simulink model "second_24_02_25_FRANCO"  (R2024a)
settings: Solver=VariableStepAuto  StartTime=0.0  StopTime=inf  FixedStep=1e-3  MaxStep=100e-6  RelTol=0.1e-3
values from neighbouring files (symbols this model uses):
  f = 5000    [second_parameters.m]
  l = 10e-3    (= 0.01)    [second_parameters.m]
  phi = atan(f*2*pi*l/r)    [second_parameters.m]
  r = 10    [second_parameters.m]
  z = sqrt(r^2+(2*pi*f*l)^2)    [second_parameters.m]
libraries: simulink x4, simulink_extras x1
settings Model: Creator=claudio.rossi  LastModifiedBy=s0001205361
settings OptimizationCC: ReuseModelBlockBuffer=off
settings RTWCC: GPUComputeCapability=3.5

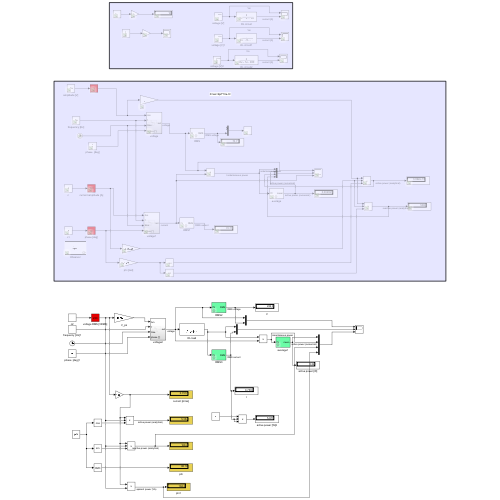
[thumbnail: Simulink's stored preview of the top-level diagram]
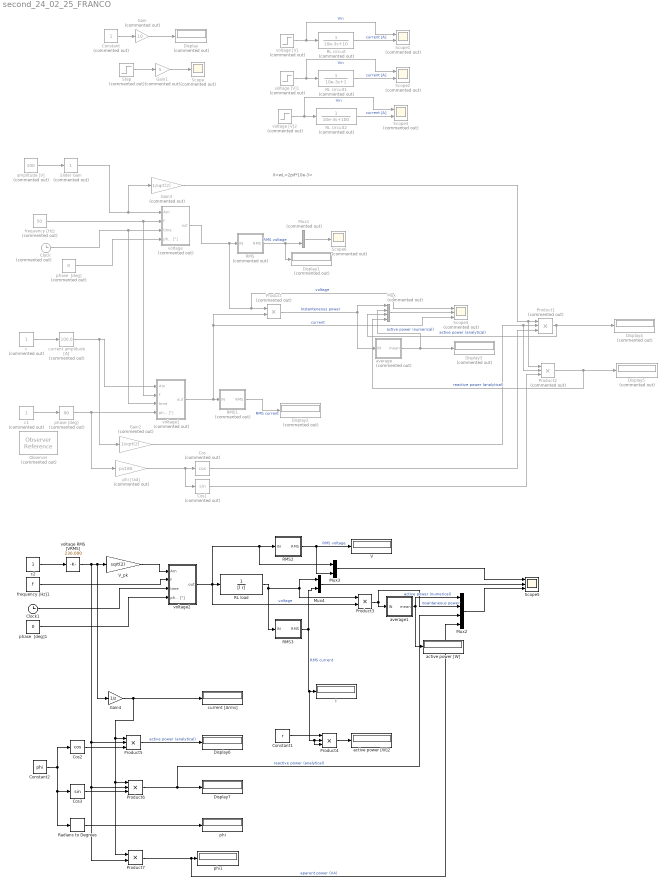
== system second_24_02_25_FRANCO ==
  note: X=wL=2pif*10e-3=
  Clock : Clock  Commented=on
  Clock1 : Clock
  Constant : Constant  Commented=on
  Constant1 : Constant  Value=r
  Constant2 : Constant  Value=phi
  Cos : Trigonometry  Commented=on  Operator=cos
  Cos1 : Trigonometry  Commented=on
  Cos2 : Trigonometry  Operator=cos
  Cos3 : Trigonometry
  Display{,1..5} (6 alike) : Display  Commented=on
  Display6 : Display
  Display7 : Display
  Gain : Gain  Commented=on  Gain=10
  Gain1 : Gain  Commented=on  Gain=5
  Gain2 : Gain  Commented=on  Gain=1/sqrt(2)
  Gain3 : Gain  Commented=on  Gain=1/sqrt(2)
  Gain4 : Gain  Gain=1/z
  I : Display
  Mux : Mux  Commented=on
  Mux1 : Mux  Commented=on  Inputs=2
  Mux2 : Mux
  Mux3 : Mux  Inputs=2
  Mux4 : Mux  Inputs=2
  Observer : ObserverReference  Commented=on  ObserverModelName=second_24_02_25_FRANCO_Observer1
  Product : Product  Commented=on
  Product1 : Product  Commented=on  Inputs=3
  Product2 : Product  Commented=on  Inputs=3
  Product3 : Product
  Product4 : Product  Inputs=3
  Product5 : Product  Inputs=3
  Product6 : Product  Inputs=3
  Product7 : Product
  RL circuit : TransferFcn  Commented=on  Denominator=[10e-3 10]
  RL circuit1 : TransferFcn  Commented=on  Denominator=[10e-3 1]
  RL circuit2 : TransferFcn  Commented=on  Denominator=[10e-3 100]
  RL load : TransferFcn  Denominator=[l r]
  RMS : Subsystem  Commented=on  mask{period=20e-3}
      mask prompts: period "period [s]"
      mask DialogControl DescTextVar Prompt: calculates the RMS of a periodic function with period specified here
  RMS1 : Subsystem  Commented=on  mask{period=20e-3}
      mask prompts: period "period [s]"
      mask DialogControl DescTextVar Prompt: calculates the RMS of a periodic function with period specified here
  RMS2 : Subsystem  mask{period=1/f}
      mask prompts: period "period [s]"
      mask DialogControl DescTextVar Prompt: calculates the RMS of a periodic function with period specified here
  RMS3 : Subsystem  mask{period=1/f}
      mask prompts: period "period [s]"
      mask DialogControl DescTextVar Prompt: calculates the RMS of a periodic function with period specified here
  Radians to Degrees : simulink_extras/Transformations/Radians to Degrees
  Scope : Scope  Commented=on
  Scope1 : Scope  Commented=on  NumInputPorts=2
  Scope2 : Scope  Commented=on  NumInputPorts=2
  Scope3 : Scope  Commented=on  NumInputPorts=2
  Scope4 : Scope  Commented=on  NumInputPorts=3
  Scope5 : Scope  NumInputPorts=3
  Scope6 : Scope  Commented=on
  Slider Gain : simulink/Math Operations/Slider Gain  Commented=on  gain=1  low=0  high=2
  Step : Step  Commented=on  SampleTime=0
  V : Display
  V_pk : Gain  Gain=sqrt(2)
  active power [W] : Display
  active power [W]2 : Display
  amplitude [V] : Constant  Commented=on  Value=100
  average : Subsystem  Commented=on  mask{period=20}
      mask prompts: period "period [s]"
  average1 : Subsystem  mask{period=20}
      mask prompts: period "period [s]"
  c : Constant  Commented=on
  c1 : Constant  Commented=on
  c2 : Constant
  current [Arms] : Display
  current amplitude [A] : simulink/Math Operations/Slider Gain  Commented=on  gain=100.0  low=0  high=100
  frequency [Hz] : Constant  Commented=on  Value=50
  frequency [Hz]1 : Constant  Value=f
  phase  [deg] : Constant  Commented=on  Value=0
  phase  [deg]1 : Constant  Value=0
  phase [deg] : simulink/Math Operations/Slider Gain  Commented=on  gain=90  low=-180  high=180
  phi : Display
  phi [rad] : Gain  Commented=on  Gain=pi/180
  phi1 : Display
  voltage : Subsystem  Commented=on
  voltage RMS [VRMS] : simulink/Math Operations/Slider Gain  gain=230.000  low=0  high=230
  voltage [V] : Step  Commented=on  After=100  SampleTime=0
  voltage [V]1 : Step  Commented=on  After=100  SampleTime=0
  voltage [V]2 : Step  Commented=on  After=100  SampleTime=0
  voltage1 : Subsystem  Commented=on
  voltage2 : Subsystem
  wires:
  Constant/1 -> Gain/1
  Step/1 -> Gain1/1
  Gain/1 -> Display/1
  Gain1/1 -> Scope/1
  voltage [V]/1 -> Scope1/1, RL circuit/1  "Vin"
  RL circuit/1 -> Scope1/2  "current [A]"
  RL circuit1/1 -> Scope2/2  "current [A]"
  voltage [V]1/1 -> RL circuit1/1, Scope2/1  "Vin"
  voltage [V]2/1 -> Scope3/1, RL circuit2/1  "Vin"
  RL circuit2/1 -> Scope3/2  "current [A]"
  amplitude [V]/1 -> Slider Gain/1
  frequency [Hz]/1 -> voltage1/2(f), voltage/2(f)
  Clock/1 -> voltage1/3(time), voltage/3(time)
  phase  [deg]/1 -> voltage/4(phase [°])
  voltage/1(out) -> Scope4/1, Product/1, RMS/1(IN)  "voltage"
  Slider Gain/1 -> Gain3/1, voltage/1(Am)
  Mux1/1 -> Scope6/1
  RMS/1(RMS) -> Display1/1, Mux1/2  "RMS voltage"
  current amplitude [A]/1 -> Gain2/1, voltage1/1(Am)
  c1/1 -> phase [deg]/1
  c/1 -> current amplitude [A]/1
  phase [deg]/1 -> phi [rad]/1, voltage1/4(phase [°])
  voltage1/1(out) -> Scope4/3, Product/2, RMS1/1(IN)  "current"
  RMS1/1(RMS) -> Display2/1  "RMS current"
  Product/1 -> average/1(IN), Mux/1  "Instanteneous power"
  average/1(mean) -> Mux/2, Display3/1  "active power (numerical)"
  Mux/1 -> Scope4/2
  Gain3/1 -> Product2/1, Product1/1
  Gain2/1 -> Product2/2, Product1/2
  phi [rad]/1 -> Cos1/1, Cos/1
  Cos/1 -> Product1/3
  Product1/1 -> Mux/3, Display4/1  "active power (analytical)"
  Product2/1 -> Mux/4, Display5/1  "reactive power (analytical)"
  Cos1/1 -> Product2/3
  voltage RMS [VRMS]/1 -> V_pk/1, Gain4/1, Product7/2, Product6/2, Product5/2
  phase  [deg]1/1 -> voltage2/4(phase [°])
  Clock1/1 -> voltage2/3(time)
  frequency [Hz]1/1 -> voltage2/2(f)
  c2/1 -> voltage RMS [VRMS]/1
  V_pk/1 -> voltage2/1(Am)
  voltage2/1(out) -> Product3/2, Mux3/1, RMS2/1(IN), RL load/1  "voltage"
  RL load/1 -> RMS3/1(IN), Product3/1, Mux4/1
  Mux2/1 -> Scope5/3
  RMS2/1(RMS) -> Mux3/2, V/1  "RMS voltage"
  RMS3/1(RMS) -> Mux4/2, Product4/3, Product4/2, I/1  "RMS current"
  Mux3/1 -> Scope5/1
  Mux4/1 -> Scope5/2
  Product3/1 -> Mux2/2, average1/1(IN)  "insantaneous power"
  average1/1(mean) -> Mux2/1, active power [W]/1  "active power (numerical)"
  Constant1/1 -> Product4/1
  Product4/1 -> active power [W]2/1
  Product6/1 -> Mux2/3, Display7/1  "reactive power (analytical)"
  Product5/1 -> Display6/1  "active power (analytical)"
  Gain4/1 -> Product5/1, Product7/1, Product6/1, current [Arms]/1
  Cos2/1 -> Product5/3
  Cos3/1 -> Product6/3
  Constant2/1 -> Radians to Degrees/1, Cos3/1, Cos2/1
  Radians to Degrees/1 -> phi/1
  Product7/1 -> Mux2/4, phi1/1  "aparent power (VA)"

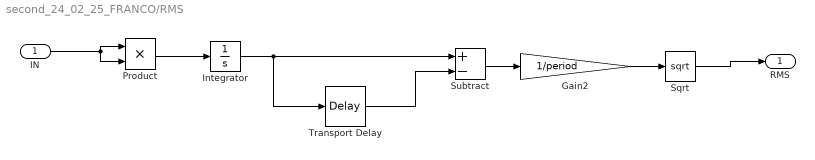
== system second_24_02_25_FRANCO/RMS ==
  IN : Inport
  Gain2 : Gain  Gain=1/period
  Integrator : Integrator
  Product : Product
  Sqrt : Sqrt
  Subtract : Sum  Inputs=+-
  Transport Delay : TransportDelay  DelayTime=period
  RMS : Outport
  wires:
  Transport Delay/1 -> Subtract/2
  Subtract/1 -> Gain2/1
  Integrator/1 -> Subtract/1, Transport Delay/1
  IN/1 -> Product/1, Product/2
  Product/1 -> Integrator/1
  Gain2/1 -> Sqrt/1
  Sqrt/1 -> RMS/1

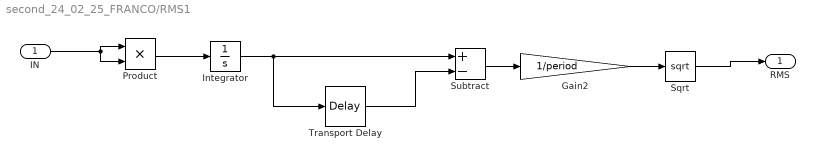
== system second_24_02_25_FRANCO/RMS1 ==
  IN : Inport
  Gain2 : Gain  Gain=1/period
  Integrator : Integrator
  Product : Product
  Sqrt : Sqrt
  Subtract : Sum  Inputs=+-
  Transport Delay : TransportDelay  DelayTime=period
  RMS : Outport
  wires:
  Sqrt/1 -> RMS/1
  Gain2/1 -> Sqrt/1
  Product/1 -> Integrator/1
  IN/1 -> Product/2, Product/1
  Integrator/1 -> Transport Delay/1, Subtract/1
  Subtract/1 -> Gain2/1
  Transport Delay/1 -> Subtract/2

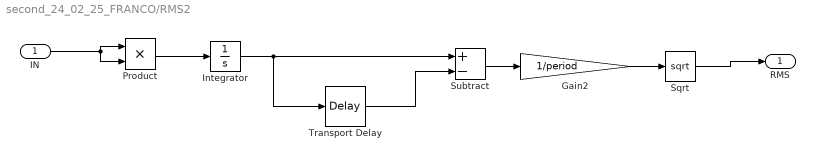
== system second_24_02_25_FRANCO/RMS2 ==
  IN : Inport
  Gain2 : Gain  Gain=1/period
  Integrator : Integrator
  Product : Product
  Sqrt : Sqrt
  Subtract : Sum  Inputs=+-
  Transport Delay : TransportDelay  DelayTime=period
  RMS : Outport
  wires:
  Sqrt/1 -> RMS/1
  Gain2/1 -> Sqrt/1
  Product/1 -> Integrator/1
  IN/1 -> Product/2, Product/1
  Integrator/1 -> Transport Delay/1, Subtract/1
  Subtract/1 -> Gain2/1
  Transport Delay/1 -> Subtract/2

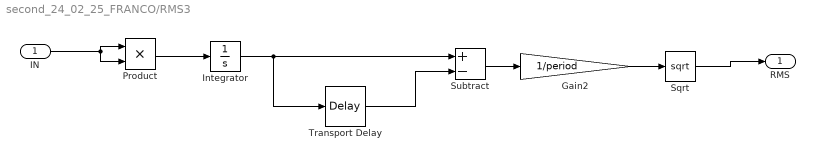
== system second_24_02_25_FRANCO/RMS3 ==
  IN : Inport
  Gain2 : Gain  Gain=1/period
  Integrator : Integrator
  Product : Product
  Sqrt : Sqrt
  Subtract : Sum  Inputs=+-
  Transport Delay : TransportDelay  DelayTime=period
  RMS : Outport
  wires:
  Transport Delay/1 -> Subtract/2
  Subtract/1 -> Gain2/1
  Integrator/1 -> Subtract/1, Transport Delay/1
  IN/1 -> Product/1, Product/2
  Product/1 -> Integrator/1
  Gain2/1 -> Sqrt/1
  Sqrt/1 -> RMS/1

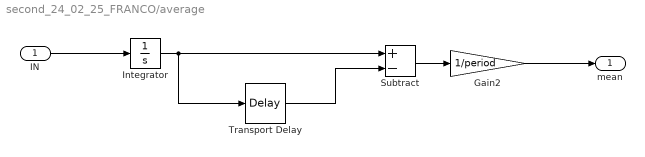
== system second_24_02_25_FRANCO/average ==
  IN : Inport
  Gain2 : Gain  Gain=1/period
  Integrator : Integrator
  Subtract : Sum  Inputs=+-
  Transport Delay : TransportDelay  DelayTime=period
  mean : Outport
  wires:
  IN/1 -> Integrator/1
  Transport Delay/1 -> Subtract/2
  Subtract/1 -> Gain2/1
  Gain2/1 -> mean/1
  Integrator/1 -> Subtract/1, Transport Delay/1

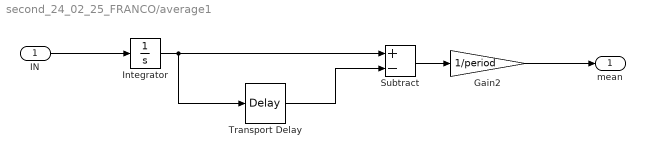
== system second_24_02_25_FRANCO/average1 ==
  IN : Inport
  Gain2 : Gain  Gain=1/period
  Integrator : Integrator
  Subtract : Sum  Inputs=+-
  Transport Delay : TransportDelay  DelayTime=period
  mean : Outport
  wires:
  Integrator/1 -> Transport Delay/1, Subtract/1
  Gain2/1 -> mean/1
  Subtract/1 -> Gain2/1
  Transport Delay/1 -> Subtract/2
  IN/1 -> Integrator/1

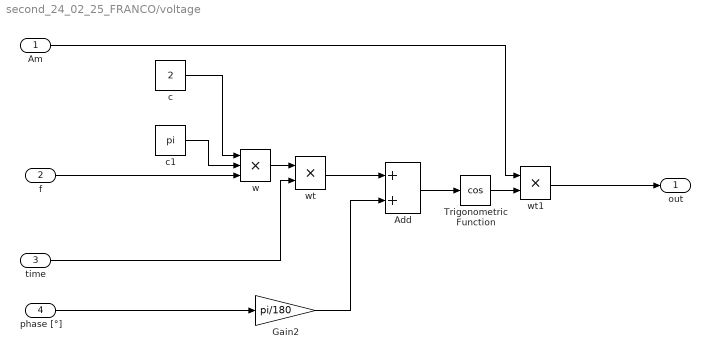
== system second_24_02_25_FRANCO/voltage ==
  Am : Inport
  f : Inport  Port=2
  time : Inport  Port=3
  phase [°] : Inport  Port=4
  Add : Sum
  Gain2 : Gain  Gain=pi/180
  Trigonometric Function : Trigonometry  Operator=cos
  c : Constant  Value=2
  c1 : Constant  Value=pi
  w : Product  Inputs=3
  wt : Product
  wt1 : Product
  out : Outport
  wires:
  wt/1 -> Add/1
  Add/1 -> Trigonometric Function/1
  phase [°]/1 -> Gain2/1
  c/1 -> w/1
  w/1 -> wt/1
  Trigonometric Function/1 -> wt1/2
  c1/1 -> w/2
  Gain2/1 -> Add/2
  wt1/1 -> out/1
  f/1 -> w/3
  time/1 -> wt/2
  Am/1 -> wt1/1

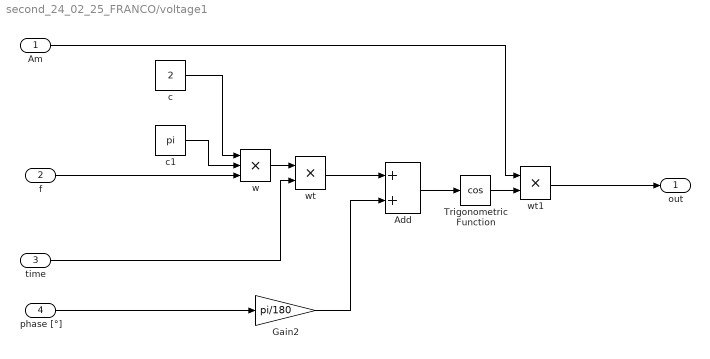
== system second_24_02_25_FRANCO/voltage1 ==
  Am : Inport
  f : Inport  Port=2
  time : Inport  Port=3
  phase [°] : Inport  Port=4
  Add : Sum
  Gain2 : Gain  Gain=pi/180
  Trigonometric Function : Trigonometry  Operator=cos
  c : Constant  Value=2
  c1 : Constant  Value=pi
  w : Product  Inputs=3
  wt : Product
  wt1 : Product
  out : Outport
  wires:
  Am/1 -> wt1/1
  time/1 -> wt/2
  f/1 -> w/3
  wt1/1 -> out/1
  Gain2/1 -> Add/2
  c1/1 -> w/2
  Trigonometric Function/1 -> wt1/2
  w/1 -> wt/1
  c/1 -> w/1
  phase [°]/1 -> Gain2/1
  Add/1 -> Trigonometric Function/1
  wt/1 -> Add/1

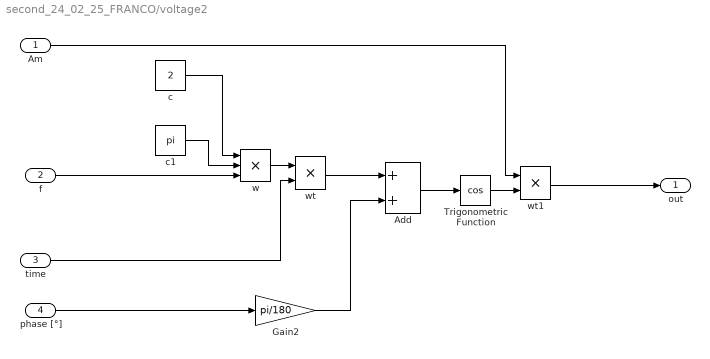
== system second_24_02_25_FRANCO/voltage2 ==
  Am : Inport
  f : Inport  Port=2
  time : Inport  Port=3
  phase [°] : Inport  Port=4
  Add : Sum
  Gain2 : Gain  Gain=pi/180
  Trigonometric Function : Trigonometry  Operator=cos
  c : Constant  Value=2
  c1 : Constant  Value=pi
  w : Product  Inputs=3
  wt : Product
  wt1 : Product
  out : Outport
  wires:
  Am/1 -> wt1/1
  time/1 -> wt/2
  f/1 -> w/3
  wt1/1 -> out/1
  Gain2/1 -> Add/2
  c1/1 -> w/2
  Trigonometric Function/1 -> wt1/2
  w/1 -> wt/1
  c/1 -> w/1
  phase [°]/1 -> Gain2/1
  Add/1 -> Trigonometric Function/1
  wt/1 -> Add/1
